simulink model "untitled1"  (R2024a)
settings: Solver=FixedStepAuto  StartTime=0.0  StopTime=5  FixedStep=0.001  RelTol=1e-3
settings Model: Creator=ventus  LastModifiedBy=ventus

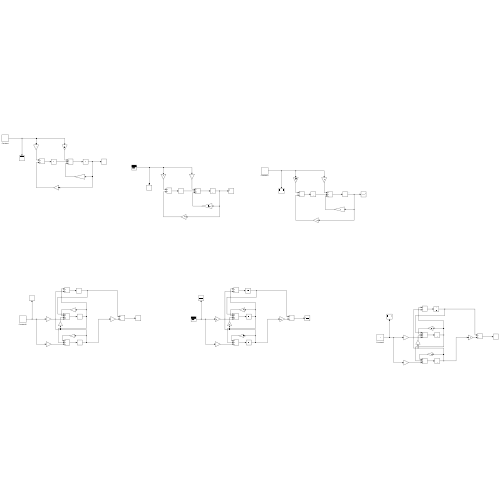
[thumbnail: Simulink's stored preview of the top-level diagram]
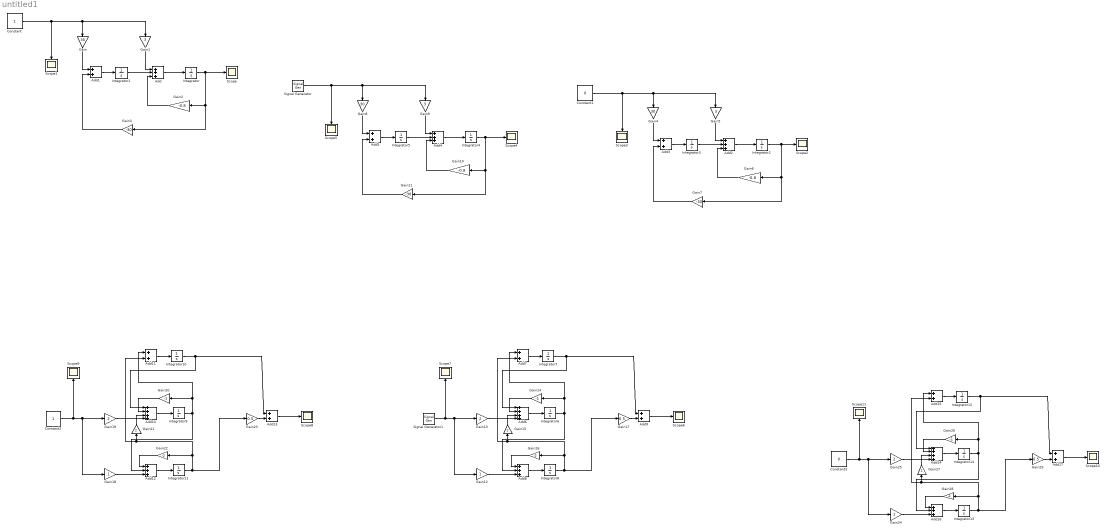
== system untitled1 ==
  Add{,2,4,8,12,16} (6 alike) : Sum  Inputs=+++
  Add{1,3,5,7,9,11,13,15,17} (9 alike) : Sum
  Add10 : Sum  Inputs=++++
  Add14 : Sum  Inputs=++++
  Add6 : Sum  Inputs=++++
  Constant : Constant  VectorParams1D=off  SampleTime=-1
  Constant1 : Constant  Value=0  VectorParams1D=off  SampleTime=-1
  Constant2 : Constant  VectorParams1D=off  SampleTime=-1
  Constant3 : Constant  Value=0  VectorParams1D=off  SampleTime=-1
  Gain : Gain  Gain=30
  Gain1 : Gain  Gain=3
  Gain10 : Gain  Gain=-0.8
  Gain11 : Gain  Gain=-30
  Gain12 : Gain
  Gain{13,15,19,21,25,27} (6 alike) : Gain  Gain=2
  Gain14 : Gain  Gain=-1
  Gain16 : Gain  Gain=-2
  Gain17 : Gain  Gain=0.5
  Gain18 : Gain
  Gain2 : Gain  Gain=-0.8
  Gain20 : Gain  Gain=-1
  Gain22 : Gain  Gain=-2
  Gain23 : Gain  Gain=0.5
  Gain24 : Gain
  Gain26 : Gain  Gain=-1
  Gain28 : Gain  Gain=-2
  Gain29 : Gain  Gain=0.5
  Gain3 : Gain  Gain=-30
  Gain4 : Gain  Gain=30
  Gain5 : Gain  Gain=3
  Gain6 : Gain  Gain=-0.8
  Gain7 : Gain  Gain=-30
  Gain8 : Gain  Gain=30
  Gain9 : Gain  Gain=3
  Integrator{,1,4..11,13} (11 alike) : Integrator
  Integrator12 : Integrator  InitialCondition=0.5
  Integrator14 : Integrator  InitialCondition=-2
  Integrator2 : Integrator  InitialCondition=1
  Integrator3 : Integrator  InitialCondition=1.3
  Scope{,1..11} (12 alike) : Scope
  Signal Generator : SignalGenerator  Amplitude=2  Units=rad/sec
  Signal Generator1 : SignalGenerator  Amplitude=2  Units=rad/sec
  wires:
  Constant/1 -> Gain/1, Gain1/1, Scope1/1
  Gain1/1 -> Add/1
  Gain/1 -> Add1/1
  Add/1 -> Integrator/1
  Integrator/1 -> Gain3/1, Gain2/1, Scope/1
  Gain2/1 -> Add/3
  Integrator1/1 -> Add/2
  Gain3/1 -> Add1/2
  Add1/1 -> Integrator1/1
  Constant1/1 -> Scope3/1, Gain4/1, Gain5/1
  Gain6/1 -> Add2/3
  Gain4/1 -> Add3/1
  Add3/1 -> Integrator3/1
  Gain7/1 -> Add3/2
  Integrator2/1 -> Gain7/1, Gain6/1, Scope2/1
  Gain5/1 -> Add2/1
  Integrator3/1 -> Add2/2
  Add2/1 -> Integrator2/1
  Add5/1 -> Integrator5/1
  Gain11/1 -> Add5/2
  Add4/1 -> Integrator4/1
  Integrator4/1 -> Gain11/1, Gain10/1, Scope4/1
  Gain8/1 -> Add5/1
  Integrator5/1 -> Add4/2
  Signal Generator/1 -> Scope5/1, Gain8/1, Gain9/1
  Gain9/1 -> Add4/1
  Gain10/1 -> Add4/3
  Gain26/1 -> Add14/2
  Gain27/1 -> Add14/3
  Add15/1 -> Integrator12/1
  Integrator12/1 -> Add14/1, Add17/1
  Gain29/1 -> Add17/2
  Gain25/1 -> Add14/4
  Integrator14/1 -> Add16/2, Add15/1, Gain26/1
  Integrator13/1 -> Gain29/1, Gain28/1, Add15/2, Gain27/1
  Gain28/1 -> Add16/1
  Constant3/1 -> Scope11/1, Gain25/1, Gain24/1
  Add14/1 -> Integrator14/1
  Gain24/1 -> Add16/3
  Add16/1 -> Integrator13/1
  Add17/1 -> Scope10/1
  Add7/1 -> Integrator7/1
  Integrator7/1 -> Add6/1, Add9/1
  Gain14/1 -> Add6/2
  Gain15/1 -> Add6/3
  Gain13/1 -> Add6/4
  Add8/1 -> Integrator8/1
  Gain12/1 -> Add8/3
  Add6/1 -> Integrator6/1
  Gain16/1 -> Add8/1
  Add9/1 -> Scope6/1
  Integrator8/1 -> Gain17/1, Gain16/1, Add7/2, Gain15/1
  Integrator6/1 -> Add8/2, Add7/1, Gain14/1
  Gain17/1 -> Add9/2
  Signal Generator1/1 -> Scope7/1, Gain13/1, Gain12/1
  Constant2/1 -> Scope9/1, Gain19/1, Gain18/1
  Gain18/1 -> Add12/3
  Integrator11/1 -> Gain23/1, Gain22/1, Add11/2, Gain21/1
  Add13/1 -> Scope8/1
  Gain22/1 -> Add12/1
  Add10/1 -> Integrator9/1
  Gain23/1 -> Add13/2
  Integrator9/1 -> Add12/2, Add11/1, Gain20/1
  Add12/1 -> Integrator11/1
  Gain19/1 -> Add10/4
  Add11/1 -> Integrator10/1
  Gain20/1 -> Add10/2
  Gain21/1 -> Add10/3
  Integrator10/1 -> Add10/1, Add13/1
